simulink model "mysimulink"  (R2014a)
settings: Solver=ode45  StartTime=0.0  StopTime=10.0  RelTol=1e-3
settings Model: Creator=gxnuhuang  LastModifiedBy=gxnuhuang
settings DataIOCC: ExternalInput=[t,u],[t,t]  LoadExternalInput=on  TimeSaveName=tou  OutputSaveName=you

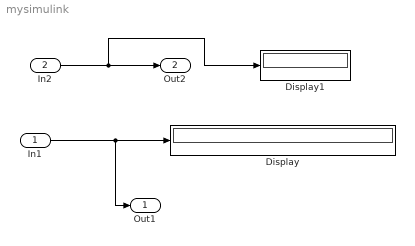
== system mysimulink ==
  In1 : Inport
  In2 : Inport  Port=2
  Display : Display
  Display1 : Display
  Out1 : Outport
  Out2 : Outport  Port=2  OutMax=[5]
  wires:
  In1/1 -> Out1/1, Display/1
  In2/1 -> Display1/1, Out2/1
